simulink model "CIE_337_Part_B_Sine"  (R2018b)
settings: Solver=FixedStepAuto  StartTime=0.0  StopTime=0.01  FixedStep=0.000001  RelTol=1e-3
libraries: simulink x1
settings Model: Creator=RAWN  LastModifiedBy=RAWN

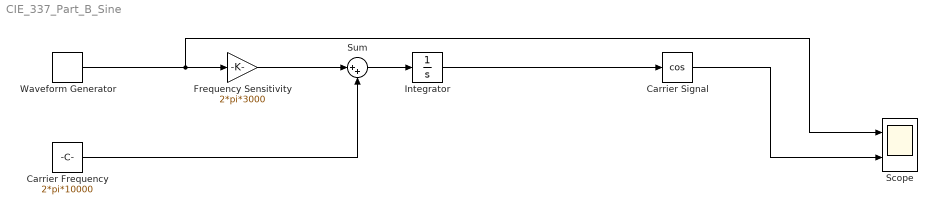
== system CIE_337_Part_B_Sine ==
  Carrier Frequency : Constant  Value=2*pi*10000
  Carrier Signal : Trigonometry  Operator=cos
  Frequency Sensitivity : Gain  Gain=2*pi*3000
  Integrator : Integrator
  Scope : Scope  NumInputPorts=2
  Sum : Sum  Inputs=|++
  Waveform Generator : simulink/Sources/Waveform Generator  OutMin=[]  OutMax=[]  OutDataTypeStr=double  SelectedSignal=1  Signals=sin('Amplitude', 1.5, 'Frequency', 2*pi*2000, 'Phase', 0)  BlockNames=MultiportSwitch_ee9397c68065416  SampleTime=0.000001
      settings: SourceProductName=Simulink
  wires:
  Sum/1 -> Integrator/1
  Waveform Generator/1 -> Scope/1, Frequency Sensitivity/1
  Integrator/1 -> Carrier Signal/1
  Carrier Frequency/1 -> Sum/2
  Frequency Sensitivity/1 -> Sum/1
  Carrier Signal/1 -> Scope/2
